simulink model "Task11_3_5"  (R2021a)
settings: Solver=VariableStepAuto  StartTime=0.0  StopTime=T  RelTol=1e-3
values from neighbouring files (symbols this model uses):
  A = [5 3 ... (first row only)    [T_5.m]
  B = [0 ... (first row only)    [T_5.m]
  C = [5 0]    [T_5.m]
  D = 6    [T_5.m]
  Gamma_f = [0 1 ... (first row only)    [T_5.m]
  H_f = [1 0]    [T_5.m]
  K = -H/M    [T_5.m]
  Lf = double([s.lf1 s.lf2])    [T_5.m]
  xif_0 = double([xi_f_1(0); xi_f_2(0)])    [T_5.m]
settings Model: Creator=fedor  LastModifiedBy=fedor

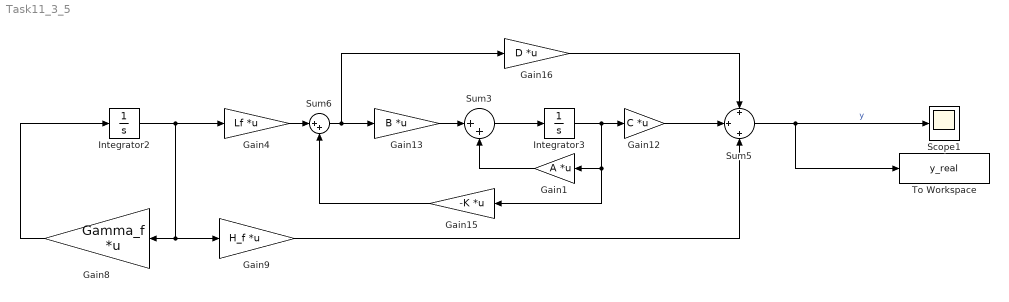
== system Task11_3_5 ==
  Gain1 : Gain  Gain=A  Multiplication=Matrix(K*u)
  Gain12 : Gain  Gain=C  Multiplication=Matrix(K*u)
  Gain13 : Gain  Gain=B  Multiplication=Matrix(K*u)
  Gain15 : Gain  Gain=-K  Multiplication=Matrix(K*u)
  Gain16 : Gain  Gain=D  Multiplication=Matrix(K*u)
  Gain4 : Gain  Gain=Lf  Multiplication=Matrix(K*u)
  Gain8 : Gain  Gain=Gamma_f  Multiplication=Matrix(K*u)
  Gain9 : Gain  Gain=H_f  Multiplication=Matrix(K*u)
  Integrator2 : Integrator  InitialCondition=xif_0
  Integrator3 : Integrator
  Scope1 : Scope
  Sum3 : Sum  Inputs=|++
  Sum5 : Sum  Inputs=+|+|+
  Sum6 : Sum  Inputs=|++
  To Workspace : ToWorkspace  VariableName=y_real  SaveFormat=Structure With Time  SampleTime=0.01
  wires:
  Integrator2/1 -> Gain9/1, Gain8/1, Gain4/1
  Gain8/1 -> Integrator2/1
  Gain13/1 -> Sum3/1
  Gain12/1 -> Sum5/2
  Gain16/1 -> Sum5/1
  Integrator3/1 -> Gain15/1, Gain1/1, Gain12/1
  Gain15/1 -> Sum6/2
  Sum3/1 -> Integrator3/1
  Sum6/1 -> Gain16/1, Gain13/1
  Gain4/1 -> Sum6/1
  Sum5/1 -> To Workspace/1, Scope1/1  "y"
  Gain1/1 -> Sum3/2
  Gain9/1 -> Sum5/3
